simulink model "HW04_Problem1"  (R2014a)
settings: Solver=ode3  StartTime=0.0  StopTime=50  FixedStep=0.001  RelTol=1e-3
settings Model: Creator=kothmann  LastModifiedBy=kothmann
settings DataIOCC: SignalLoggingSaveFormat=ModelDataLogs
settings OptimizationCC: ExpressionDepthLimit=2147483647
settings DebuggingCC: UnderspecifiedInitializationDetection=Classic  FcnCallInpInsideContextMsg=EnableAllAsWarning  StateNameClashWarn=warning
settings GRTTargetCC: CombineOutputUpdateFcns=off  GRTInterface=on

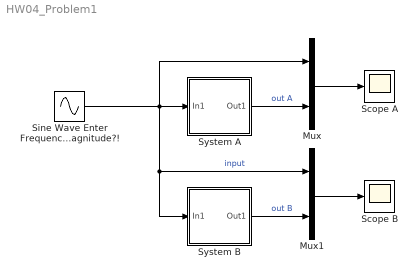
== system HW04_Problem1 ==
  Mux : Mux  Inputs=2
  Mux1 : Mux  Inputs=2
  Scope A : Scope
      settings: ShowLegends=on
  Scope B : Scope
      settings: ShowLegends=on
  Sine Wave Enter Frequency in Here What About Magnitude?! : Sin  Amplitude=2  Frequency=4  SampleTime=0
  System A : Subsystem
  System B : Subsystem
  wires:
  Sine Wave Enter Frequency in Here What About Magnitude?!/1 -> Mux/1, System A/1(In1), System B/1(In1), Mux1/1  "input"
  System A/1(Out1) -> Mux/2  "out A"
  Mux/1 -> Scope A/1
  System B/1(Out1) -> Mux1/2  "out B"
  Mux1/1 -> Scope B/1

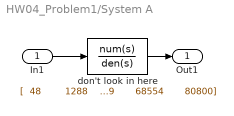
== system HW04_Problem1/System A ==
  In1 : Inport
  don't look in here : TransferFcn  Numerator="[  48        1288        9760       32400       40000]"  Denominator="[6         161        1431        7629       27899       68554       80800]"
  Out1 : Outport
  wires:
  In1/1 -> don't look in here/1
  don't look in here/1 -> Out1/1

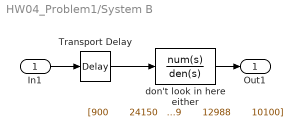
== system HW04_Problem1/System B ==
  In1 : Inport
  Transport Delay : TransportDelay  DelayTime=0.0000000025E8
  don't look in here either : TransferFcn  Numerator="[900       24150      183000      607500      750000]"  Denominator="[ 6         167        1490        6329       12988       10100]"
  Out1 : Outport
  wires:
  don't look in here either/1 -> Out1/1
  In1/1 -> Transport Delay/1
  Transport Delay/1 -> don't look in here either/1
